simulink library "NeuroMuscularLibrary"  (R2019b)
settings: Solver=ode45  StartTime=0.0  StopTime=10.0  RelTol=1e-3  EnableMultiTasking=on
values from neighbouring files (symbols this model uses):
  a_18_19 = 116    [Prosthesis3R60Params.m]
  a_18_21 = 34    [Prosthesis3R60Params.m]
  a_2_3 = 18    [Prosthesis3R60Params.m]
  angle_offset = 0    [Prosthesis3R60Params.m]
  ankle_height = 0.08    [BodyMechParams.m]
  c = 0.05    [BodyMechParams.m]
  c_jointstop = 0.3 / (pi/180)    (= 17.1887338539)    [BodyMechParams.m]
  c_stance_comp_a0 = 885.0653    [Prosthesis3R60Params.m]
  c_stance_comp_a1 = 2.1443    [Prosthesis3R60Params.m]
  cg14 = 1/2*L14    (= 0.0475)    [Prosthesis3R60Params.m]
  cg25 = (5.45/11.05)*L25    (= 0.0379527149321)    [Prosthesis3R60Params.m]
  cg3 = (3.6/10.4)*L3    (= 0.0306346153846)    [Prosthesis3R60Params.m]
  d_fBall = 0.1    [BodyMechParams.m]
  d_fHeel = 0.05    [BodyMechParams.m]
  deltaLegAngleThr = 8*pi/180    (= 0.13962634016)    [CMGParams.m]
  DeltaThRef = 2e-3    (= 0.002)    [BodyMechParams.m]
  dt_visual = 0.001    [Prosthesis3R60Params.m]
  eref = 0.04    [BodyMechParams.m]
  Fmax = 4000    [MuscleEnergyTest.m]
  FmaxGLU = 1500    [BodyMechParams.m]
  footBallToAnkleDist = 0.16    [BodyMechParams.m]
  footBallToCenterDist = footLength/2    (= 0.1)    [BodyMechParams.m]
  footBallToHeelDist = footLength    (= 0.2)    [BodyMechParams.m]
  footCenterToCGDist = 0.14 - footBallToCenterDist    (= 0.04)    [BodyMechParams.m]
  footInertia = 0.005    [BodyMechParams.m]
  footLength = 0.2    [BodyMechParams.m]
  footMass = 1.25    [BodyMechParams.m]
  FT = 20    [MuscleEnergyTest.m]
  FT_GLU = 47.6    [BodyMechParams.m]
  g = 9.80665    [BodyMechParams.m]
  groundTheta = [atan(diff(groundZ)./diff(groundX)), 0]    [generateGround.m]
  groundZ = groundZ * stepSize/(largestStep+eps)    [generateGround.m]
  hatCenterToCGDist = 0.35 - hatHipToCenterDistLen    (= -0.05)    [BodyMechParams.m]
  hatHipToCenterDistLen = hatLength/2    (= 0.4)    [BodyMechParams.m]
  hatInertia = 3    [BodyMechParams.m]
  hatLeftHipToCenterDistWidth = .15    (= 0.15)    [BodyMechParams.m]
  hatLength = 0.8    [BodyMechParams.m]
  hatMass = 53.5    [BodyMechParams.m]
  hatThickness = 0.2    [BodyMechParams.m]
  hatWidth = 0.4    [BodyMechParams.m]
  J1011 = (4130)*1e-9    (= 4.13e-06)    [Prosthesis3R60Params.m]
  J1415 = (1.18*1e5)*1e-9    (= 0.000118)    [Prosthesis3R60Params.m]
  J18192021 = (6.86*1e4)*1e-9    (= 6.86e-05)    [Prosthesis3R60Params.m]
  J2526 = (3.59*1e4)*1e-9    (= 3.59e-05)    [Prosthesis3R60Params.m]
  J3467 = (25.96*1e4)*1e-9    (= 0.0002596)    [Prosthesis3R60Params.m]
  K = 5    [BodyMechParams.m]
  k_gn = k_gn/2    (= 39226.6)    [BodyMechParams.m]
  k_gt = k_gt/2    (= 39226.6)    [BodyMechParams.m]
  k_pressure = hatMass * g / DeltaThRef    (= 262327.8875)    [BodyMechParams.m]
  k_stance = 130000    [Prosthesis3R60Params.m]
  k_swing = 18750    [Prosthesis3R60Params.m]
  L0_stance = 0.08925    [Prosthesis3R60Params.m]
  L0_swing = 0.0896    [Prosthesis3R60Params.m]
  L10 = 7.9*1e-3    (= 0.0079)    [Prosthesis3R60Params.m]
  L11 = 3.3*1e-3    (= 0.0033)    [Prosthesis3R60Params.m]
  L14 = 95*1e-3    (= 0.095)    [Prosthesis3R60Params.m]
  L15 = 8.2*1e-3    (= 0.0082)    [Prosthesis3R60Params.m]
  L18 = 25.1*1e-3    (= 0.0251)    [Prosthesis3R60Params.m]
  L19 = 17.7*1e-3    (= 0.0177)    [Prosthesis3R60Params.m]
  L20 = 26*1e-3    (= 0.026)    [Prosthesis3R60Params.m]
  L21 = 1.7*1e-3    (= 0.0017)    [Prosthesis3R60Params.m]
  L25 = 76.95*1e-3    (= 0.07695)    [Prosthesis3R60Params.m]
  L26 = 2.8*1e-3    (= 0.0028)    [Prosthesis3R60Params.m]
  L3 = 88.5*1e-3    (= 0.0885)    [Prosthesis3R60Params.m]
  L4 = 1.7*1e-3    (= 0.0017)    [Prosthesis3R60Params.m]
  L6 = 40.25*1e-3    (= 0.04025)    [Prosthesis3R60Params.m]
  L7 = 14.9*1e-3    (= 0.0149)    [Prosthesis3R60Params.m]
  leg_l = [(thighLength - ankle_height/2) (shankLength - ankle_height/2)]    [BodyMechParams.m]
  legAngleSpeedMax = 10    [CMGParams.m]
  lopt = 0.055    [MuscleEnergyTest.m]
  loptBFSH = 0.12    [BodyMechParams.m]
  loptGAS = 0.05    [BodyMechParams.m]
  loptGLU = 0.11    [BodyMechParams.m]
  loptHAB = 0.09    [BodyMechParams.m]
  loptHAD = 0.10    (= 0.1)    [BodyMechParams.m]
  loptHAM = 0.10    (= 0.1)    [BodyMechParams.m]
  loptHFL = 0.11    [BodyMechParams.m]
  loptRF = 0.08    [BodyMechParams.m]
  loptSOL = 0.04    [BodyMechParams.m]
  loptTA = 0.06    [BodyMechParams.m]
  loptVAS = 0.08    [BodyMechParams.m]
  lslack = 0.245    [MuscleEnergyTest.m]
  lslackBFSH = 0.10    (= 0.1)    [BodyMechParams.m]
  lslackGAS = 0.40    (= 0.4)    [BodyMechParams.m]
  lslackGLU = 0.13    [BodyMechParams.m]
  lslackHAB = 0.07    [BodyMechParams.m]
  lslackHAD = 0.18    [BodyMechParams.m]
  lslackHAM = 0.31    [BodyMechParams.m]
  lslackHFL = 0.10    (= 0.1)    [BodyMechParams.m]
  lslackRF = 0.35    [BodyMechParams.m]
  lslackSOL = 0.26    [BodyMechParams.m]
  lslackTA = 0.24    [BodyMechParams.m]
  lslackVAS = 0.23    [BodyMechParams.m]
  m1011 = 49.5*1e-3    (= 0.0495)    [Prosthesis3R60Params.m]
  m1415 = 123.8*1e-3    (= 0.1238)    [Prosthesis3R60Params.m]
  m18192021 = 196.6*1e-3    (= 0.1966)    [Prosthesis3R60Params.m]
  m2526 = 58.3*1e-3    (= 0.0583)    [Prosthesis3R60Params.m]
  m3467 = 253.3*1e-3    (= 0.2533)    [Prosthesis3R60Params.m]
  mu_slide = 0.8    [BodyMechParams.m]
  mu_stick = 0.9    [BodyMechParams.m]
  N = 1.5    [BodyMechParams.m]    (also in cmaes.m = size(x,1); mergeCompareEnergyCosts.m = {S.name})
  phiKneeUpLimit = 5*pi/180    (= 0.0872664625997)    [BodyMechParams.m]
  phimaxGASa = (100-90)*pi/180    (= 0.174532925199)    [BodyMechParams.m]
  phimaxGASk = (180-140)*pi/180    (= 0.698131700798)    [BodyMechParams.m]
  phimaxRFk = (180-165)*pi/180    (= 0.261799387799)    [BodyMechParams.m]
  phimaxSOL = (100-90)*pi/180    (= 0.174532925199)    [BodyMechParams.m]
  phimaxTA = (80-90)*pi/180    (= -0.174532925199)    [BodyMechParams.m]
  phimaxVAS = (180-165)*pi/180    (= 0.261799387799)    [BodyMechParams.m]
  phirefBFSH = (180-160)*pi/180    (= 0.349065850399)    [BodyMechParams.m]
  phirefGASa = (80-90)*pi/180    (= -0.174532925199)    [BodyMechParams.m]
  phirefGASk = (180-165)*pi/180    (= 0.261799387799)    [BodyMechParams.m]
  phirefGLU = (120-180)*pi/180    (= -1.0471975512)    [BodyMechParams.m]
  phirefHAB = 10*pi/180    (= 0.174532925199)    [BodyMechParams.m]
  phirefHAD = 15*pi/180    (= 0.261799387799)    [BodyMechParams.m]
  phirefHAMh = (150-180)*pi/180    (= -0.523598775598)    [BodyMechParams.m]
  phirefHAMk = (180-180)*pi/180    (= 0)    [BodyMechParams.m]
  phirefHFL = (160-180)*pi/180    (= -0.349065850399)    [BodyMechParams.m]
  phirefRFh = (170-180)*pi/180    (= -0.174532925199)    [BodyMechParams.m]
  phirefRFk = (180-125)*pi/180    (= 0.959931088597)    [BodyMechParams.m]
  phirefSOL = (90-90)*pi/180    (= 0)    [BodyMechParams.m]
  ... (+64 more)
undefined symbols (not defined in the file or in its folder): ankleBackDriveGain, ankleCJointstop, ankleDgain, ankleFilterPID, ankleFilterSEA, ankleGearEff, ankleGearRatio, ankleIgain, ankleInitialAngle, ankleInputMass, ankleIntCoulomb, ankleIntDamping, ankleIntStatic, ankleParallelSpringDamping, ankleParallelSpringOffset, ankleParallelSpringStiffness, anklePgain, anklePlantarLimit, ankleSEADamping, ankleSEAStiffness, ankleTendonMass, ankleWMaxJointstop, D12_F, D12_S, D12_T, D12z_T, D13_F, D1G_F, D1G_HAT, D1G_S, D1G_T, D1Gy_F, DeltaS, DeltaSGLU, DeltaSHFL, dryFrictionDamping, dryFrictionStiffness, dryFrictionVelThresh, footMassp, FourBarL1, FourBarL3, GainDphiHATGLUst, GainDphiHATHABst, GainDphiHATHADst, GainDphiHATHFLst, GainFGASst, GainFGLUst, GainFHABst, GainFHAMst, GainFSOLst, GainFSOLTAst, GainFVASst, GainGAS, GainGLU, GainGLUswing, GainHAM, GainHAMHFL ... (+194)
libraries: sm_lib x332, nesl_utility x156, simulink x33, dspswit3 x30, $bdroot x19, simulink_extras x7
(part 14 of 15)

== system NeuroMuscularLibrary/RMHeel Cnt/3D Contact ==
  RefPt [m m m] : Inport
  nVec [m m m] : Inport  Port=2
  pVec [m m m] : Inport  Port=3
  vVec [m/s m/s m/s] : Inport  Port=4
  Contact! : EnablePort  StatesWhenEnabling=reset
  Friction Switch : Subsystem
  Kinetic Friction Model : Subsystem
  Logical Operator : Logic  Operator=NOT  AllPortsSameDT=off  OutDataTypeStr=boolean
  Static Friction Model : Subsystem
  Sum : Sum
  Sum1 : Sum
  FnVec [N N N] : Outport  OutputWhenDisabled=reset  InitialOutput=[0 0 0]
      settings: AttributesFormatString=when disabled: %<OutputWhenDisabled>
  FtVec [N N N] : Outport  Port=2  OutputWhenDisabled=reset  InitialOutput=[0 0 0]
      settings: AttributesFormatString=when disabled: %<OutputWhenDisabled>
  wires:
  pVec [m m m]/1 -> Static Friction Model/1(pos [m]), Kinetic Friction Model/2(pos [m m m])
  vVec [m/s m/s m/s]/1 -> Kinetic Friction Model/1(vel [m/s m/s m/s]), Static Friction Model/2(vel [m/s m/s m/s])
  Kinetic Friction Model/2(posFP [m m m]) -> Static Friction Model/4(posFP [m])
  Friction Switch/1(Stiction) -> Static Friction Model/Enable, Logical Operator/1
  Logical Operator/1 -> Kinetic Friction Model/Enable
  nVec [m m m]/1 -> Kinetic Friction Model/4(nVec [m m m])
  Kinetic Friction Model/4(Stiction!) -> Friction Switch/2(Stick!)
  Static Friction Model/1(F_n Stick [N N N]) -> Sum1/1
  Kinetic Friction Model/6(F_n Slide [N N N]) -> Sum1/2
  Kinetic Friction Model/5(F_t Slide [N N N]) -> Sum/2
  Static Friction Model/2(F_t Stick [N N N]) -> Sum/1
  Sum1/1 -> FnVec [N N N]/1  "F_nVec"
  Sum/1 -> FtVec [N N N]/1  "F_tVec"
  Static Friction Model/3(Sliding!) -> Friction Switch/1(Slide!)
  RefPt [m m m]/1 -> Kinetic Friction Model/3(RefPt [m m m])
  Kinetic Friction Model/3(nVec FP [m m m]) -> Static Friction Model/5(nVecFP [m m m])
  Kinetic Friction Model/1(RefPtFP [m m m]) -> Static Friction Model/3(RefPtFP [m m m])

== system NeuroMuscularLibrary/Swing Phase/Filtered Derivative ==
  In1 : Inport
  Filter Coeff : Gain  Gain=legAngleFilter
  Integrator : Integrator
  Sum4 : Sum  Inputs=|+-
  Out1 : Outport
  wires:
  Integrator/1 -> Sum4/2
  Sum4/1 -> Filter Coeff/1
  Filter Coeff/1 -> Integrator/1, Out1/1
  In1/1 -> Sum4/1

== system NeuroMuscularLibrary/Swing Phase/Knee Flex ==
  LegAngleSpeed : Inport
  Enable : EnablePort  StatesWhenEnabling=reset  ZeroCross=off
  " 4" : Gain  Gain=-kneeFlexGain
  Saturation : Saturate  UpperLimit=0  LowerLimit=-inf  ZeroCross=off
  tau : Outport  OutputWhenDisabled=reset  InitialOutput=0
  wires:
  LegAngleSpeed/1 -> Saturation/1
  " 4"/1 -> tau/1
  Saturation/1 -> " 4"/1

== system NeuroMuscularLibrary/Swing Phase/Knee Hold ==
  legAngleSpeed : Inport
  legAngle : Inport  Port=2
  legAngleTgt : Inport  Port=3
  kneeSpeed : Inport  Port=4
  Enable : EnablePort  StatesWhenEnabling=reset  ZeroCross=off
  " 5" : Gain  Gain=-kneeHoldGain1
  " 6" : Gain  Gain=-kneeHoldGain2
  Add4 : Sum
  Compare To Zero : simulink/Logic and Bit Operations/Compare To Zero  relop=>=  OutDataTypeStr=boolean  ZeroCross=off
  Compare To Zero1 : simulink/Logic and Bit Operations/Compare To Zero  relop=<  OutDataTypeStr=boolean  ZeroCross=off
  Product1 : Product
  Product2 : Product  Inputs=5
  Relational Operator : RelationalOperator  Operator=<  OutDataTypeStr=boolean  ZeroCross=off  RndMeth=Nearest
  Saturation : Saturate  UpperLimit=inf  LowerLimit=0
  Sum1 : Sum  Inputs=+-|
  Sum3 : Sum  Inputs=+-|
  tau : Outport  OutputWhenDisabled=reset  InitialOutput=0
  wires:
  Product1/1 -> Add4/1
  Saturation/1 -> Add4/2
  Add4/1 -> tau/1
  legAngleTgt/1 -> Sum1/2
  legAngle/1 -> Sum1/1
  legAngleSpeed/1 -> Relational Operator/2, Sum3/1
  Product2/1 -> Saturation/1
  Compare To Zero1/1 -> Product2/4
  Sum3/1 -> Product2/3
  Sum1/1 -> Product2/2
  " 6"/1 -> Product2/1
  kneeSpeed/1 -> Relational Operator/1, Compare To Zero1/1, Sum3/2, Compare To Zero/1, " 5"/1, " 6"/1  "knee speed"
  Compare To Zero/1 -> Product1/2
  " 5"/1 -> Product1/1
  Relational Operator/1 -> Product2/5

== system NeuroMuscularLibrary/Swing Phase/Knee Stop ==
  note: Knee Extend Torque
  legAngleSpeed : Inport
  legAngle : Inport  Port=2
  legAngleTgt : Inport  Port=3
  Leg Length : Inport  Port=4
  Extend? : Inport  Port=5
  Enable : EnablePort  StatesWhenEnabling=reset  ZeroCross=off
  Add : Sum
  Add5 : Sum  Inputs=-+
  Add6 : Sum  Inputs=+-
  Constant10 : Constant
  Constant11 : Constant  Value=legAngleSpeedMax
  Constant12 : Constant  Value=-kneeExtendGain
  Constant13 : Constant  Value=shankLength + thighLength
  Constant9 : Constant  Value=kneeStopGain
  Divide : Product  Inputs=*/
  Divide1 : Product  Inputs=***
  Product4 : Product  Inputs=5
  Relational Operator1 : RelationalOperator  Operator=<  OutDataTypeStr=boolean  ZeroCross=off  RndMeth=Nearest
  Relational Operator2 : RelationalOperator  Operator=<  OutDataTypeStr=boolean  ZeroCross=off  RndMeth=Nearest
  Sum2 : Sum  Inputs=++|
  Sum5 : Sum  Inputs=|-+
  leg angle Threshold : Constant  Value=deltaLegAngleThr
  tau : Outport  OutputWhenDisabled=reset  InitialOutput=0
  wires:
  Extend?/1 -> Divide1/1
  Leg Length/1 -> Sum5/1
  legAngleSpeed/1 -> Divide/1, Relational Operator2/1
  legAngle/1 -> Add5/1, Relational Operator1/1
  legAngleTgt/1 -> Sum2/1
  Add/1 -> tau/1
  Divide1/1 -> Add/2
  Sum5/1 -> Divide1/3
  Constant13/1 -> Sum5/2
  Constant12/1 -> Divide1/2
  Product4/1 -> Add/1
  Relational Operator2/1 -> Product4/5
  Relational Operator1/1 -> Product4/4
  Divide/1 -> Add6/2
  Constant10/1 -> Add6/1
  Add6/1 -> Product4/2
  Constant11/1 -> Divide/2, Relational Operator2/2
  Constant9/1 -> Product4/3
  Add5/1 -> Product4/1
  Sum2/1 -> Relational Operator1/2, Add5/2
  leg angle Threshold/1 -> Sum2/2

== system NeuroMuscularLibrary/Swing Phase/Wait 100 ms to enable ==
  In1 : Inport
  Clock : Clock
  Compare To Constant : simulink/Logic and Bit Operations/Compare To Constant  relop=>  const=.1  OutDataTypeStr=boolean  ZeroCross=off
  Product6 : Product
  Out1 : Outport
  wires:
  Product6/1 -> Out1/1
  Clock/1 -> Compare To Constant/1
  Compare To Constant/1 -> Product6/1
  In1/1 -> Product6/2

== system NeuroMuscularLibrary/Swing Phase (sagittal)/kneei_flexion from alpha ==
  note: Knee Phase i
  SBFSH : Inport
  Enable : EnablePort  StatesWhenEnabling=reset  ZeroCross=off
  SBFSH_Sw_ki : Outport  OutputWhenDisabled=reset  InitialOutput=0
  wires:
  SBFSH/1 -> SBFSH_Sw_ki/1

== system NeuroMuscularLibrary/Swing Phase (sagittal)/kneeii_damp and hold &kneeiii_leg stop &kneeiv_stance preparation ==
  note: Knee Phase i
  Target Leg Angle : Inport
  LceRF : Inport  Port=2
  LceHAM : Inport  Port=3
  VceHAM : Inport  Port=4
  VceVAS : Inport  Port=5
  VceBFSH : Inport  Port=6
  VceRF : Inport  Port=7
  LceHFL : Inport  Port=8
  LceGLU : Inport  Port=9
  LceVAS : Inport  Port=10
  Enable : EnablePort  StatesWhenEnabling=reset  ZeroCross=off
  " 1" : Gain  Gain=Sw_a2lopt_HAM
  " 9" : Gain  Gain=Sw_a2lopt_RF
  Compare To Constant : simulink/Logic and Bit Operations/Compare To Constant  relop=<=  const=0  OutDataTypeStr=uint8  ZeroCross=off
  Constant1 : Constant  Value=0  OutDataTypeStr=boolean
  Constant10 : Constant  Value=Sw_aRef_HAM
  Constant2 : Constant  Value=0  OutDataTypeStr=boolean
  Constant3 : Constant  Value=0  OutDataTypeStr=boolean
  Constant4 : Constant
  Constant5 : Constant
  Constant6 : Constant  Value=deltaLegAngleThr
  Constant8 : Constant  Value=Sw_aRef_RF
  Logical Operator : Logic  Operator=NOT  AllPortsSameDT=off  OutDataTypeStr=boolean
  Logical Operator1 : Logic  AllPortsSameDT=off  OutDataTypeStr=boolean
  Relational Operator : RelationalOperator  Operator=<=  OutDataTypeStr=boolean  ZeroCross=off  RndMeth=Nearest
  Relational Operator1 : RelationalOperator  OutDataTypeStr=boolean  ZeroCross=off  RndMeth=Nearest
  S-R Flip-Flop : simulink_extras/Flip Flops/S-R Flip-Flop  initial_condition=0
  S-R Flip-Flop1 : simulink_extras/Flip Flops/S-R Flip-Flop  initial_condition=0
  S-R Flip-Flop2 : simulink_extras/Flip Flops/S-R Flip-Flop  initial_condition=0
  Sum1 : Sum  Inputs=+-|  SaturateOnIntegerOverflow=on  InputSameDT=on  OutDataTypeStr=Inherit: Same as first input
  Sum2 : Sum  Inputs=++|  SaturateOnIntegerOverflow=on  InputSameDT=on  OutDataTypeStr=Inherit: Same as first input
  Sum3 : Sum  Inputs=|+-  SaturateOnIntegerOverflow=on  InputSameDT=on  OutDataTypeStr=Inherit: Same as first input
  Sum4 : Sum  Inputs=+-|  SaturateOnIntegerOverflow=on  InputSameDT=on  OutDataTypeStr=Inherit: Same as first input
  Sum5 : Sum  Inputs=++|  SaturateOnIntegerOverflow=on  InputSameDT=on  OutDataTypeStr=Inherit: Same as first input
  Terminator : Terminator
  Terminator1 : Terminator
  Terminator2 : Terminator
  kneeii_damp and hold : Subsystem  TreatAsAtomicUnit=on
  kneeiii_leg stop : Subsystem  TreatAsAtomicUnit=on
  kneeiv_stance preparation : Subsystem  TreatAsAtomicUnit=on
  SRF_Sw_kii : Outport  OutputWhenDisabled=reset  InitialOutput=0
  SBFSH_Sw_kii : Outport  Port=2  OutputWhenDisabled=reset  InitialOutput=0
  SHAM_Sw_kiii : Outport  Port=3  OutputWhenDisabled=reset  InitialOutput=0
  SBFSH_Sw_kiii : Outport  Port=4  OutputWhenDisabled=reset  InitialOutput=0
  SGAS_Sw_kiii : Outport  Port=5  OutputWhenDisabled=reset  InitialOutput=0
  SHFL_Sw_kiv : Outport  Port=6  OutputWhenDisabled=reset  InitialOutput=0
  SGLU_Sw_kiv : Outport  Port=7  OutputWhenDisabled=reset  InitialOutput=0
  SVAS_Sw_kiv : Outport  Port=8  OutputWhenDisabled=reset  InitialOutput=0
  wires:
  Constant1/1 -> S-R Flip-Flop/2
  S-R Flip-Flop/2 -> Terminator/1
  Relational Operator/1 -> S-R Flip-Flop/1
  Constant2/1 -> S-R Flip-Flop1/2
  S-R Flip-Flop1/2 -> Terminator1/1
  Relational Operator1/1 -> S-R Flip-Flop1/1
  Constant3/1 -> S-R Flip-Flop2/2
  S-R Flip-Flop2/2 -> Terminator2/1
  Logical Operator1/1 -> S-R Flip-Flop2/1
  S-R Flip-Flop/1 -> Logical Operator/1
  S-R Flip-Flop1/1 -> kneeiii_leg stop/Enable, Logical Operator1/1
  S-R Flip-Flop2/1 -> kneeiv_stance preparation/Enable
  kneeii_damp and hold/1(SRF_Sw_kii) -> SRF_Sw_kii/1
  kneeii_damp and hold/2(SBFSH_Sw_kii) -> SBFSH_Sw_kii/1
  kneeiii_leg stop/1(SHAM_Sw_kiii) -> SHAM_Sw_kiii/1
  kneeiii_leg stop/2(SBFSH_Sw_kiii) -> SBFSH_Sw_kiii/1
  kneeiii_leg stop/3(SGAS_Sw_kiii) -> SGAS_Sw_kiii/1
  kneeiv_stance preparation/1(SHFL_Sw_kiv) -> SHFL_Sw_kiv/1
  kneeiv_stance preparation/2(SGLU_Sw_kiv) -> SGLU_Sw_kiv/1
  kneeiv_stance preparation/3(SVAS_Sw_kiv) -> SVAS_Sw_kiv/1
  Sum3/1 -> " 9"/1
  Constant4/1 -> Sum5/2
  " 9"/1 -> Sum5/1
  Target Leg Angle/1 -> kneeiv_stance preparation/1(Target Leg Angle), kneeiii_leg stop/1(Target Leg Angle), kneeii_damp and hold/1(Target Leg Angle), Sum3/1, Sum2/1
  Sum5/1 -> Relational Operator/2  "lceOffRF"
  LceRF/1 -> Relational Operator/1, kneeii_damp and hold/5(LceRF)
  Logical Operator/1 -> kneeii_damp and hold/Enable
  Sum2/1 -> Sum1/1  "a_thr"
  Sum1/1 -> " 1"/1
  Constant5/1 -> Sum4/1
  " 1"/1 -> Sum4/2
  Sum4/1 -> Relational Operator1/2  "lceOffHAM"
  LceHAM/1 -> kneeiii_leg stop/2(LceHAM), Relational Operator1/1  "LceHAM"
  Compare To Constant/1 -> Logical Operator1/2
  VceHAM/1 -> Compare To Constant/1
  VceBFSH/1 -> kneeii_damp and hold/3(VceBFSH)
  VceRF/1 -> kneeii_damp and hold/4(VceRF)
  LceHFL/1 -> kneeiv_stance preparation/2(LceHFL)
  LceGLU/1 -> kneeiv_stance preparation/3(LceGLU)
  LceVAS/1 -> kneeiv_stance preparation/4(LceVAS)
  VceVAS/1 -> kneeii_damp and hold/2(VceVAS)
  Constant10/1 -> Sum1/2
  Constant6/1 -> Sum2/2
  Constant8/1 -> Sum3/2

== system NeuroMuscularLibrary/Swing Phase Hip muscle/Filtered Derivative ==
  In1 : Inport
  Filter Coeff : Gain  Gain=legAngleFilter
  Integrator : Integrator
  Sum4 : Sum  Inputs=|+-
  Out1 : Outport
  wires:
  In1/1 -> Sum4/1
  Filter Coeff/1 -> Out1/1, Integrator/1
  Sum4/1 -> Filter Coeff/1
  Integrator/1 -> Sum4/2

== system NeuroMuscularLibrary/Swing Phase Hip muscle/Knee Flex ==
  LegAngleSpeed : Inport
  Enable : EnablePort  StatesWhenEnabling=reset  ZeroCross=off
  " 4" : Gain  Gain=-kneeFlexGain
  Saturation : Saturate  UpperLimit=0  LowerLimit=-inf  ZeroCross=off
  tau : Outport  OutputWhenDisabled=reset  InitialOutput=0
  wires:
  Saturation/1 -> " 4"/1
  " 4"/1 -> tau/1
  LegAngleSpeed/1 -> Saturation/1

== system NeuroMuscularLibrary/Swing Phase Hip muscle/Knee Hold ==
  legAngleSpeed : Inport
  legAngle : Inport  Port=2
  legAngleTgt : Inport  Port=3
  kneeSpeed : Inport  Port=4
  Enable : EnablePort  StatesWhenEnabling=reset  ZeroCross=off
  " 5" : Gain  Gain=-kneeHoldGain1
  " 6" : Gain  Gain=-kneeHoldGain2
  Add4 : Sum
  Compare To Zero : simulink/Logic and Bit Operations/Compare To Zero  relop=>=  OutDataTypeStr=boolean  ZeroCross=off
  Compare To Zero1 : simulink/Logic and Bit Operations/Compare To Zero  relop=<  OutDataTypeStr=boolean  ZeroCross=off
  Product1 : Product
  Product2 : Product  Inputs=5
  Relational Operator : RelationalOperator  Operator=<  OutDataTypeStr=boolean  ZeroCross=off  RndMeth=Nearest
  Saturation : Saturate  UpperLimit=inf  LowerLimit=0
  Sum1 : Sum  Inputs=+-|
  Sum3 : Sum  Inputs=+-|
  tau : Outport  OutputWhenDisabled=reset  InitialOutput=0
  wires:
  Relational Operator/1 -> Product2/5
  " 5"/1 -> Product1/1
  Compare To Zero/1 -> Product1/2
  kneeSpeed/1 -> " 6"/1, " 5"/1, Compare To Zero/1, Sum3/2, Compare To Zero1/1, Relational Operator/1  "knee speed"
  " 6"/1 -> Product2/1
  Sum1/1 -> Product2/2
  Sum3/1 -> Product2/3
  Compare To Zero1/1 -> Product2/4
  Product2/1 -> Saturation/1
  legAngleSpeed/1 -> Sum3/1, Relational Operator/2
  legAngle/1 -> Sum1/1
  legAngleTgt/1 -> Sum1/2
  Add4/1 -> tau/1
  Saturation/1 -> Add4/2
  Product1/1 -> Add4/1

== system NeuroMuscularLibrary/Swing Phase Hip muscle/Knee Stop ==
  note: Knee Extend Torque
  legAngleSpeed : Inport
  legAngle : Inport  Port=2
  legAngleTgt : Inport  Port=3
  Leg Length : Inport  Port=4
  Extend? : Inport  Port=5
  Enable : EnablePort  StatesWhenEnabling=reset  ZeroCross=off
  Add : Sum
  Add5 : Sum  Inputs=-+
  Add6 : Sum  Inputs=+-
  Constant10 : Constant
  Constant11 : Constant  Value=legAngleSpeedMax
  Constant12 : Constant  Value=-kneeExtendGain
  Constant13 : Constant  Value=shankLength + thighLength
  Constant9 : Constant  Value=kneeStopGain
  Divide : Product  Inputs=*/
  Divide1 : Product  Inputs=***
  Product4 : Product  Inputs=5
  Relational Operator1 : RelationalOperator  Operator=<  OutDataTypeStr=boolean  ZeroCross=off  RndMeth=Nearest
  Relational Operator2 : RelationalOperator  Operator=<  OutDataTypeStr=boolean  ZeroCross=off  RndMeth=Nearest
  Sum2 : Sum  Inputs=++|
  Sum5 : Sum  Inputs=|-+
  leg angle Threshold : Constant  Value=deltaLegAngleThr
  tau : Outport  OutputWhenDisabled=reset  InitialOutput=0
  wires:
  leg angle Threshold/1 -> Sum2/2
  Sum2/1 -> Add5/2, Relational Operator1/2
  Add5/1 -> Product4/1
  Constant9/1 -> Product4/3
  Constant11/1 -> Relational Operator2/2, Divide/2
  Add6/1 -> Product4/2
  Constant10/1 -> Add6/1
  Divide/1 -> Add6/2
  Relational Operator1/1 -> Product4/4
  Relational Operator2/1 -> Product4/5
  Product4/1 -> Add/1
  Constant12/1 -> Divide1/2
  Constant13/1 -> Sum5/2
  Sum5/1 -> Divide1/3
  Divide1/1 -> Add/2
  Add/1 -> tau/1
  legAngleTgt/1 -> Sum2/1
  legAngle/1 -> Relational Operator1/1, Add5/1
  legAngleSpeed/1 -> Relational Operator2/1, Divide/1
  Leg Length/1 -> Sum5/1
  Extend?/1 -> Divide1/1

== system NeuroMuscularLibrary/Swing Phase Hip muscle/Wait 100 ms to enable ==
  In1 : Inport
  Clock : Clock
  Compare To Constant : simulink/Logic and Bit Operations/Compare To Constant  relop=>  const=.1  OutDataTypeStr=boolean  ZeroCross=off
  Product6 : Product
  Out1 : Outport
  wires:
  In1/1 -> Product6/2
  Compare To Constant/1 -> Product6/1
  Clock/1 -> Compare To Constant/1
  Product6/1 -> Out1/1

== system NeuroMuscularLibrary/ThighSong/Sensor Sheet ==
  note: Inner Segment Pressure Sheet
  FB Gain1 : Gain  Gain=1/DeltaThRef  SaturateOnIntegerOverflow=on  OutDataTypeStr=Inherit: Same as input  ParamDataTypeStr=Inherit: Same as input
  Gain1 : Gain  Gain=-1
  Gain3 : Gain  Gain=k_pressure
  Gain4 : Gain  Gain=1/v_max_pressure
  Mux1 : Mux  Inputs=2
  PS-Simulink Converter : nesl_utility/PS-Simulink Converter  PhysicalDomain=network_engine_domain  SubClassName=ps_output  LeftPortType=input  RightPortType=output  PseudoPeriodic=off  Frequencies=[]  Unit=1  AffineConversion=off
  PS-Simulink Converter1 : nesl_utility/PS-Simulink Converter  PhysicalDomain=network_engine_domain  SubClassName=ps_output  LeftPortType=input  RightPortType=output  PseudoPeriodic=off  Frequencies=[]  Unit=1  AffineConversion=off
  Pressure Sheet Reaction Force : Fcn  Expr=-u(1) * (1+sgn(u(1))*u(2))
  Prismatic Joint : sm_lib/Joints/Prismatic Joint  JointMode=Normal  SenseConstraintForce=off  SenseConstraintForceX=off  SenseConstraintForceY=off  SenseConstraintForceZ=off  SenseConstraintTorque=off  SenseConstraintTorqueX=off  SenseConstraintTorqueY=off  SenseConstraintTorqueZ=off  SenseTotalForce=off  SenseTotalForceX=off  SenseTotalForceY=off  SenseTotalForceZ=off  SenseTotalTorque=off  SenseTotalTorqueX=off  SenseTotalTorqueY=off  SenseTotalTorqueZ=off  CompositeWrenchDir=FollowerOnBase  CompositeWrenchFrame=BaseFrame  EquilibriumPosition=0  EquilibriumPositionUnits=m  SpringStiffness=0  SpringStiffnessUnits=N/m  DampingCoefficient=0  DampingCoefficientUnits=N/(m/s)  TorqueActuationMode=InputTorque  MotionActuationMode=ComputedMotion  SensePosition=on  SenseVelocity=on  SenseAcceleration=off  SenseTorqueForce=off  SenseLowerLimitTorqueForce=off  SenseUpperLimitTorqueForce=off  LowerLimitSpecify=off  LowerLimitBound=-1  LowerLimitBoundUnits=m  LowerLimitStiffness=1e6  LowerLimitStiffnessUnits=N/m  LowerLimitDamping=1e3  LowerLimitDampingUnits=N/(m/s)  LowerLimitTransitionRegionWidth=1e-4  LowerLimitTransitionRegionWidthUnits=m  UpperLimitSpecify=off  UpperLimitBound=1  UpperLimitBoundUnits=m  UpperLimitStiffness=1e6  UpperLimitStiffnessUnits=N/m  UpperLimitDamping=1e3  UpperLimitDampingUnits=N/(m/s)  UpperLimitTransitionRegionWidth=1e-4  UpperLimitTransitionRegionWidthUnits=m  PositionTargetSpecify=on  PositionTargetPriority=High  PositionTargetValue=0  PositionTargetValueUnits=m  VelocityTargetSpecify=on  VelocityTargetPriority=High  VelocityTargetValue=0  VelocityTargetValueUnits=m/s
  Saturation11 : Saturate  UpperLimit=inf  LowerLimit=0  ZeroCross=off
  Simulink-PS Converter : nesl_utility/Simulink-PS Converter  PhysicalDomain=network_engine_domain  SubClassName=ps_input  LeftPortType=input  RightPortType=output  PseudoPeriodic=off  Frequencies=[]  NoiseDistribution=none  NoiseParameters=[]  Unit=1  AffineConversion=off  FilteringAndDerivatives=zero  SimscapeFilterOrder=1  InputFilterTimeConstant=0.001  UdotUserProvided=1
  Y-up TO Z-up : sm_lib/Frames and Transforms/Rigid Transform  TranslationMethod=None  TranslationStandardOffset=0  TranslationLengthUnit=m  TranslationStandardAxis=+Z  TranslationCartesianOffset=[0 0 0]  TranslationROffset=0  TranslationROffsetUnits=m  TranslationZOffset=0  TranslationZOffsetUnits=m  TranslationThetaOffset=0  TranslationThetaOffsetUnits=deg  RotationMethod=AlignedAxes  RotationAngleUnits=deg  RotationStandardAxis=+Z  RotationAngle=0  RotationArbitraryAxis=[0 0 1]  FollAlignAxisA=+X  BaseAlignAxisA=+X  FollAlignAxisB=+Z  BaseAlignAxisB=+Y  RotationSequenceAxes=FollowerAxes  RotationSequence=XYX  RotationSequenceAngles=[0 0 0]  RotationSequenceAnglesUnits=deg  RotationMatrix=[1 0 0; 0 1 0; 0 0 1]
  Z-up TO Y-up : sm_lib/Frames and Transforms/Rigid Transform  TranslationMethod=None  TranslationStandardOffset=0  TranslationLengthUnit=m  TranslationStandardAxis=+Z  TranslationCartesianOffset=[0 0 0]  TranslationROffset=0  TranslationROffsetUnits=m  TranslationZOffset=0  TranslationZOffsetUnits=m  TranslationThetaOffset=0  TranslationThetaOffsetUnits=deg  RotationMethod=AlignedAxes  RotationAngleUnits=deg  RotationStandardAxis=+Z  RotationAngle=0  RotationArbitraryAxis=[0 0 1]  FollAlignAxisA=+X  BaseAlignAxisA=+X  FollAlignAxisB=+Y  BaseAlignAxisB=+Z  RotationSequenceAxes=FollowerAxes  RotationSequence=XYX  RotationSequenceAngles=[0 0 0]  RotationSequenceAnglesUnits=deg  RotationMatrix=[1 0 0; 0 1 0; 0 0 1]
  smooth : TransferFcn  Denominator=[0.02 1]
  Lower thigh : PMIOPort  Side=Left
  Upper thigh : PMIOPort  Port=2  Side=Right
  dx : Outport
  Thigh Fx : Outport  Port=2
  wires:
  PS-Simulink Converter/1 -> Gain1/1, Gain3/1  "position"
  PS-Simulink Converter1/1 -> Gain4/1  "velocity"
  Mux1/1 -> Pressure Sheet Reaction Force/1
  Gain3/1 -> Mux1/1
  Gain4/1 -> Mux1/2
  Pressure Sheet Reaction Force/1 -> Simulink-PS Converter/1
  FB Gain1/1 -> Thigh Fx/1
  smooth/1 -> Saturation11/1
  Saturation11/1 -> FB Gain1/1
  Gain1/1 -> smooth/1, dx/1
  connections:
  Prismatic Joint/LConn1 -- Y-up TO Z-up/RConn1
  Prismatic Joint/RConn1 -- Z-up TO Y-up/LConn1
  Prismatic Joint/LConn2 -- Simulink-PS Converter/RConn1
  Prismatic Joint/RConn2 -- PS-Simulink Converter/LConn1
  Prismatic Joint/RConn3 -- PS-Simulink Converter1/LConn1
  Y-up TO Z-up/LConn1 -- Lower thigh/RConn1
  Upper thigh/RConn1 -- Z-up TO Y-up/RConn1

== system NeuroMuscularLibrary/Full Prosthesis/Ankle  Joint/Ankle Plantarflexion Limit ==
  note: Knee/Hip Joint Limits
  phi [rad] : Inport
  dphi [rad/s] : Inport  Port=2
  Compare To Constant : simulink/Logic and Bit Operations/Compare To Constant  relop=<  const=1.0  OutDataTypeStr=boolean  ZeroCross=off
  Compare To Zero : simulink/Logic and Bit Operations/Compare To Zero  relop=>  OutDataTypeStr=boolean  ZeroCross=off
  Constant : Constant
  Gain : Gain  Gain=-1
  Gain1 : Gain  Gain=ext
  Gain2 : Gain  Gain=-ext
  Gain3 : Gain  Gain=c_jointstop
  Gain4 : Gain  Gain=1/w_max_jointstop
  Gain5 : Gain  Gain=ext
  Product : Product  Inputs=4
  Sum : Sum  Inputs=|+-
  Sum1 : Sum  Inputs=|+-
  overextension angle : Constant  Value=phiUpLimit
  M_stop [Nm] : Outport
  wires:
  Sum/1 -> Gain3/1
  Gain1/1 -> Compare To Zero/1, Gain/1
  Gain3/1 -> Gain1/1
  dphi [rad/s]/1 -> Gain4/1
  overextension angle/1 -> Sum/2
  phi [rad]/1 -> Sum/1
  Gain4/1 -> Gain2/1
  Gain2/1 -> Compare To Constant/1, Sum1/2
  Gain5/1 -> M_stop [Nm]/1
  Constant/1 -> Sum1/1
  Gain/1 -> Product/1
  Sum1/1 -> Product/2
  Compare To Constant/1 -> Product/3
  Compare To Zero/1 -> Product/4
  Product/1 -> Gain5/1

== system NeuroMuscularLibrary/Full Prosthesis/Ankle Motor/Friction ==
  Velocity : Inport
  Abs : Abs  ZeroCross=off
  Add : Sum  Inputs=+++
  Divide : Product  Inputs=*/*
  Gain : Gain  Gain=sigma0
  Gain1 : Gain  Gain=sigma1
  Gain2 : Gain  Gain=Fv
  Gain3 : Gain  Gain=-1
  Integrator : Integrator  ZeroCross=off
  Subtract : Sum  Inputs=+-
  g(v) : Fcn  Expr=(Fc + (Fs - Fc)*exp(-(u/v_s)^2))/sigma0
  Friction Force : Outport
  wires:
  Gain2/1 -> Add/1
  Gain/1 -> Add/2
  Gain1/1 -> Add/3
  Gain3/1 -> Friction Force/1
  Add/1 -> Gain3/1
  Integrator/1 -> Gain/1, Divide/3  "z"
  g(v)/1 -> Divide/2
  Subtract/1 -> Gain1/1, Integrator/1  "dz/dt"
  Divide/1 -> Subtract/2
  Abs/1 -> Divide/1
  Velocity/1 -> Subtract/1, Abs/1, g(v)/1, Gain2/1

== system NeuroMuscularLibrary/Full Prosthesis/Ankle Motor/Motor Dynamics ==
  Voltage : Inport
  Speed : Inport  Port=2
  1/Inductance : Gain  Gain=1/motorInductance
  Add : Sum  Inputs=+--
  Integrator : Integrator
  Resistance : Gain  Gain=motorResistance
  Saturation : Saturate  UpperLimit=motorMaxCurrent  LowerLimit=-motorMaxCurrent  ZeroCross=off
  Torsional Constant : Gain  Gain=motorTorsionalConst
  back EMF : Gain  Gain=motorBackEMF
  Torque : Outport
  wires:
  Integrator/1 -> Saturation/1
  Saturation/1 -> Torsional Constant/1, Resistance/1  "Current"
  Resistance/1 -> Add/2
  back EMF/1 -> Add/3
  1/Inductance/1 -> Integrator/1  "di/dt"
  Add/1 -> 1/Inductance/1
  Speed/1 -> back EMF/1
  Torsional Constant/1 -> Torque/1  "Torque"
  Voltage/1 -> Add/1

== system NeuroMuscularLibrary/Full Prosthesis/Ankle SEA Control/4 bar ratio ==
  Ankle Input Angle : Inport
  Tendon Angle : Inport  Port=2
  Ankle Angle : Inport  Port=3
  Add : Sum  Inputs=--+
  Bias1 : Bias  Bias=-atan(16.3/81)
  Bias3 : Bias  Bias=5*pi/2
  Divide : Product  Inputs=*/
  Gain1 : Gain  Gain=-1
  Gain2 : Gain  Gain=-1
  Gain3 : Gain  Gain=-FourBarL3/FourBarL1
  Gain4 : Gain  Gain=-1
  Trigonometric Function : Trigonometry
  Trigonometric Function1 : Trigonometry
  ratio : Outport
  wires:
  Gain1/1 -> Bias3/1
  Bias1/1 -> Add/3
  Bias3/1 -> Trigonometric Function1/1, Add/2
  Ankle Angle/1 -> Gain4/1
  Gain4/1 -> Bias1/1
  Gain3/1 -> ratio/1  "4 bar ratio"
  Gain2/1 -> Add/1
  Ankle Input Angle/1 -> Gain2/1
  Add/1 -> Trigonometric Function/1
  Tendon Angle/1 -> Gain1/1
  Trigonometric Function/1 -> Divide/1
  Trigonometric Function1/1 -> Divide/2
  Divide/1 -> Gain3/1

== system NeuroMuscularLibrary/Full Prosthesis/Ankle SEA Control/Feed Forward ==
  Motor Speed : Inport
  Load Acceleration : Inport  Port=2
  Desired Actuator Torque : Inport  Port=3
  1/n : Gain  Gain=1/ankleGearRatio
  Back EMF : Gain  Gain=motorBackEMF
  Filter Coeff : Gain  Gain=ankleFilterSEA
  Integrator : Integrator
  K_b*J_m*n : Gain  Gain=ankleBackDriveGain*motorRotorInertia*ankleGearRatio
  R/K_tau : Gain  Gain=motorResistance/motorTorsionalConst
  Sum : Sum  Inputs=+-|
  Sum1 : Sum  Inputs=|+-
  Sum2 : Sum
  Computed Motor Voltage : Outport
  wires:
  Filter Coeff/1 -> Integrator/1
  Sum1/1 -> Filter Coeff/1
  Integrator/1 -> Sum1/2, K_b*J_m*n/1  "Filtered Accel"
  Load Acceleration/1 -> Sum1/1
  Back EMF/1 -> Sum/1
  Sum2/1 -> R/K_tau/1
  R/K_tau/1 -> Sum/2
  Motor Speed/1 -> Back EMF/1
  Desired Actuator Torque/1 -> 1/n/1
  1/n/1 -> Sum2/2
  K_b*J_m*n/1 -> Sum2/1
  Sum/1 -> Computed Motor Voltage/1

== system NeuroMuscularLibrary/Full Prosthesis/Knee Joint/Friction ==
  Velocity : Inport
  Abs : Abs  ZeroCross=off
  Add : Sum  Inputs=+++
  Divide : Product  Inputs=*/*
  Gain : Gain  Gain=sigma0
  Gain1 : Gain  Gain=sigma1
  Gain2 : Gain  Gain=Fv
  Gain3 : Gain  Gain=-1
  Integrator : Integrator  ZeroCross=off
  Subtract : Sum  Inputs=+-
  g(v) : Fcn  Expr=(Fc + (Fs - Fc)*exp(-(u/v_s)^2))/sigma0
  Friction Force : Outport
  wires:
  Gain2/1 -> Add/1
  Gain/1 -> Add/2
  Gain1/1 -> Add/3
  Gain3/1 -> Friction Force/1
  Add/1 -> Gain3/1
  Integrator/1 -> Gain/1, Divide/3  "z"
  g(v)/1 -> Divide/2
  Subtract/1 -> Gain1/1, Integrator/1  "dz/dt"
  Divide/1 -> Subtract/2
  Abs/1 -> Divide/1
  Velocity/1 -> Subtract/1, Abs/1, g(v)/1, Gain2/1

== system NeuroMuscularLibrary/Full Prosthesis/Knee Joint/Knee Plantarflexion Limit ==
  note: Knee/Hip Joint Limits
  phi [rad] : Inport
  dphi [rad/s] : Inport  Port=2
  Compare To Constant : simulink/Logic and Bit Operations/Compare To Constant  relop=<  const=1.0  OutDataTypeStr=boolean  ZeroCross=off
  Compare To Zero : simulink/Logic and Bit Operations/Compare To Zero  relop=>  OutDataTypeStr=boolean  ZeroCross=off
  Constant : Constant
  Gain : Gain  Gain=-1
  Gain1 : Gain  Gain=ext
  Gain2 : Gain  Gain=-ext
  Gain3 : Gain  Gain=c_jointstop
  Gain4 : Gain  Gain=1/w_max_jointstop
  Gain5 : Gain  Gain=ext
  Product : Product  Inputs=4
  Sum : Sum  Inputs=|+-
  Sum1 : Sum  Inputs=|+-
  overextension angle : Constant  Value=phiUpLimit
  M_stop [Nm] : Outport
  wires:
  Product/1 -> Gain5/1
  Compare To Zero/1 -> Product/4
  Compare To Constant/1 -> Product/3
  Sum1/1 -> Product/2
  Gain/1 -> Product/1
  Constant/1 -> Sum1/1
  Gain5/1 -> M_stop [Nm]/1
  Gain2/1 -> Sum1/2, Compare To Constant/1
  Gain4/1 -> Gain2/1
  phi [rad]/1 -> Sum/1
  overextension angle/1 -> Sum/2
  dphi [rad/s]/1 -> Gain4/1
  Gain3/1 -> Gain1/1
  Gain1/1 -> Gain/1, Compare To Zero/1
  Sum/1 -> Gain3/1

== system NeuroMuscularLibrary/Full Prosthesis/Knee Motor/Friction ==
  Velocity : Inport
  Abs : Abs  ZeroCross=off
  Add : Sum  Inputs=+++
  Divide : Product  Inputs=*/*
  Gain : Gain  Gain=sigma0
  Gain1 : Gain  Gain=sigma1
  Gain2 : Gain  Gain=Fv
  Gain3 : Gain  Gain=-1
  Integrator : Integrator  ZeroCross=off
  Subtract : Sum  Inputs=+-
  g(v) : Fcn  Expr=(Fc + (Fs - Fc)*exp(-(u/v_s)^2))/sigma0
  Friction Force : Outport
  wires:
  Gain2/1 -> Add/1
  Gain/1 -> Add/2
  Gain1/1 -> Add/3
  Gain3/1 -> Friction Force/1
  Add/1 -> Gain3/1
  Integrator/1 -> Gain/1, Divide/3  "z"
  g(v)/1 -> Divide/2
  Subtract/1 -> Gain1/1, Integrator/1  "dz/dt"
  Divide/1 -> Subtract/2
  Abs/1 -> Divide/1
  Velocity/1 -> Subtract/1, Abs/1, g(v)/1, Gain2/1

== system NeuroMuscularLibrary/Full Prosthesis/Knee Motor/Motor Dynamics ==
  Voltage : Inport
  Speed : Inport  Port=2
  1/Inductance : Gain  Gain=1/motorInductance
  Add : Sum  Inputs=+--
  Integrator : Integrator
  Resistance : Gain  Gain=motorResistance
  Saturation : Saturate  UpperLimit=motorMaxCurrent  LowerLimit=-motorMaxCurrent  ZeroCross=off
  Torsional Constant : Gain  Gain=motorTorsionalConst
  back EMF : Gain  Gain=motorBackEMF
  Torque : Outport
  wires:
  Integrator/1 -> Saturation/1
  Saturation/1 -> Torsional Constant/1, Resistance/1  "Current"
  Resistance/1 -> Add/2
  back EMF/1 -> Add/3
  1/Inductance/1 -> Integrator/1  "di/dt"
  Add/1 -> 1/Inductance/1
  Speed/1 -> back EMF/1
  Torsional Constant/1 -> Torque/1  "Torque"
  Voltage/1 -> Add/1

== system NeuroMuscularLibrary/Full Prosthesis/Knee SEA Control/Feed Forward ==
  Motor Speed : Inport
  Load Acceleration : Inport  Port=2
  Desired Torque : Inport  Port=3
  1/n : Gain  Gain=1/kneeGearRatio
  Back EMF : Gain  Gain=motorBackEMF
  Filter Coeff : Gain  Gain=kneeFilterSEA
  Integrator : Integrator
  K_b*J_m*n : Gain  Gain=kneeBackDriveGain*motorRotorInertia*kneeGearRatio
  R/K_tau : Gain  Gain=motorResistance/motorTorsionalConst
  Sum : Sum  Inputs=+-|
  Sum1 : Sum  Inputs=|+-
  Sum2 : Sum
  Computed Motor Voltage : Outport
  wires:
  Filter Coeff/1 -> Integrator/1
  Sum1/1 -> Filter Coeff/1
  Integrator/1 -> Sum1/2, K_b*J_m*n/1  "Filtered Accel"
  Load Acceleration/1 -> Sum1/1
  Back EMF/1 -> Sum/1
  Sum2/1 -> R/K_tau/1
  R/K_tau/1 -> Sum/2
  Motor Speed/1 -> Back EMF/1
  Desired Torque/1 -> 1/n/1
  1/n/1 -> Sum2/2
  K_b*J_m*n/1 -> Sum2/1
  Sum/1 -> Computed Motor Voltage/1

== system NeuroMuscularLibrary/Ground Contact Model/2D Contact/Friction Switch ==
  note: Static/Kinetic Friction Switch
  Slide! : Inport
  Stick! : Inport  Port=2
  Memory : Memory
  S-R Flip-Flop : simulink_extras/Flip Flops/S-R Flip-Flop  initial_condition=0
  Terminator : Terminator
  Stiction : Outport
  wires:
  Memory/1 -> Stiction/1
  Slide!/1 -> S-R Flip-Flop/2
  Stick!/1 -> S-R Flip-Flop/1
  S-R Flip-Flop/2 -> Terminator/1
  S-R Flip-Flop/1 -> Memory/1

== system NeuroMuscularLibrary/Ground Contact Model/2D Contact/Kinetic Friction Model ==
  note: Tangential Ground Friction
  note: Normal Ground Friction
  note: Sliding Limit Detector
  note: Footpoint Determiner
  note: Kinetic Friction Model
  vel [m/s m/s] : Inport
  pos [m m] : Inport  Port=2
  RefPt [m m] : Inport  Port=3
  nVec [m m] : Inport  Port=4
  Enable : EnablePort  StatesWhenEnabling=reset  ZeroCross=off
  Add : Sum  Inputs=-+
  Compare To Constant : simulink/Logic and Bit Operations/Compare To Constant  relop=<  const=1  OutDataTypeStr=boolean
  Constant : Constant  Value=vLimit
  Constant2 : Constant
  FixPt Relational Operator : RelationalOperator  Operator=>  OutDataTypeStr=boolean  ZeroCross=off  RndMeth=Nearest
  Gain3 : Gain  Gain=k_gn
  Gain4 : Gain  Gain=1/v_gn_max
  Memory : Memory
  Negative : simulink/Logic and Bit Operations/Compare To Zero  relop=<  OutDataTypeStr=boolean
  Product : Product  RndMeth=Zero
  Product1 : Product  RndMeth=Zero
  Product2 : Product  Inputs=3
  Scope : Scope
  Sum : Sum  Inputs=|+-
  Vector Norm : Subsystem
  d_n : DotProduct  InputSameDT=on  OutDataTypeStr=Inherit: Inherit via internal rule
  qnVec : Sum  Inputs=-+
  reverse direction : Gain  Gain=-1
  sliding friction coefficient : Gain  Gain=mu_slide
  tVec : Product  Inputs=*/  RndMeth=Zero
  v_n : DotProduct  InputSameDT=on  OutDataTypeStr=Inherit: Inherit via internal rule
  v_nVec : Product  RndMeth=Zero
  v_tVec : Sum  Inputs=-+|
  RefPtFP [m m] : Outport  InitialOutput=[0 0]
      settings: AttributesFormatString=initial = '%<InitialOutput>'\nwhen disabled = '%<OutputWhenDisabled>'
  posFP [m m] : Outport  Port=2  InitialOutput=[0 0]
      settings: AttributesFormatString=initial = '%<InitialOutput>'\nwhen disabled = '%<OutputWhenDisabled>'
  nVec FP [m m] : Outport  Port=3  InitialOutput=0
      settings: AttributesFormatString=initial = '%<InitialOutput>'\nwhen disabled = '%<OutputWhenDisabled>'
  Stiction! : Outport  Port=4  OutputWhenDisabled=reset  InitialOutput=0
      settings: AttributesFormatString=initial = '%<InitialOutput>'\nwhen disabled = '%<OutputWhenDisabled>'
  F_t Slide [N N] : Outport  Port=5  OutputWhenDisabled=reset  InitialOutput=[0 0]
      settings: AttributesFormatString=initial = '%<InitialOutput>'\nwhen disabled = '%<OutputWhenDisabled>'
  F_n Slide [N N] : Outport  Port=6  OutputWhenDisabled=reset  InitialOutput=[0 0]
      settings: AttributesFormatString=initial = '%<InitialOutput>'\nwhen disabled = '%<OutputWhenDisabled>'
  wires:
  RefPt [m m]/1 -> RefPtFP [m m]/1, qnVec/2
  qnVec/1 -> d_n/1
  pos [m m]/1 -> qnVec/1, posFP [m m]/1
  tVec/1 -> reverse direction/1
  Product1/1 -> F_n Slide [N N]/1
  reverse direction/1 -> Scope/1, Product/2
  sliding friction coefficient/1 -> Product/1
  v_nVec/1 -> v_tVec/1
  v_n/1 -> v_nVec/1, Gain4/1
  vel [m/s m/s]/1 -> v_tVec/2, v_n/2
  d_n/1 -> Gain3/1
  nVec [m m]/1 -> nVec FP [m m]/1, Product1/1, d_n/2, v_nVec/2, v_n/1
  Constant/1 -> Sum/2
  Sum/1 -> Negative/1
  Vector Norm/1(norm) -> tVec/2, Sum/1
  Product/1 -> F_t Slide [N N]/1
  Product2/1 -> Product1/2, sliding friction coefficient/1
  Gain3/1 -> Product2/1
  Gain4/1 -> Compare To Constant/1, Add/1
  Constant2/1 -> Add/2
  Compare To Constant/1 -> Product2/3
  Add/1 -> Product2/2
  v_tVec/1 -> Vector Norm/1(vec), tVec/1
  FixPt Relational Operator/1 -> Stiction!/1
  Memory/1 -> FixPt Relational Operator/2
  Negative/1 -> FixPt Relational Operator/1, Memory/1

== system NeuroMuscularLibrary/Ground Contact Model/2D Contact/Static Friction Model ==
  note: Tangential Ground Reaction Force
  note: (distance to
      | surface)
  note: Zero multiplication prevents
      | horizontal friction model from
      | oscillating between static and kinetic
      | friction when the vertical force is zero but
      | the ground level is not yet reached
      | in the upward motion
  note: Static Friction Model
  note: Stiction Limit Detector
  pos [m] : Inport
  vel [m/s m/s] : Inport  Port=2
  RefPtFP [m m] : Inport  Port=3
  posFP [m] : Inport  Port=4
  nVecFP [m m] : Inport  Port=5
  Enable : EnablePort  StatesWhenEnabling=reset  ZeroCross=off
  Abs : Abs
  Add : Sum  Inputs=-+
  Check Vertical Friction : Product  RndMeth=Zero
  Compare To Constant : simulink/Logic and Bit Operations/Compare To Constant  relop=<  const=1  OutDataTypeStr=boolean  ZeroCross=off
  Constant : Constant
  Constant1 : Constant
  D pos_n : DotProduct  InputSameDT=on  OutDataTypeStr=Inherit: Inherit via internal rule
  Dpos_nVec : Product  RndMeth=Zero
  Dpos_tVec : Sum  Inputs=|+-
  FixPt Relational Operator : RelationalOperator  Operator=>  OutDataTypeStr=boolean  ZeroCross=off  RndMeth=Nearest
  Gain : Gain  Gain=-1
  Gain1 : Gain  Gain=k_gn
  Gain2 : Gain  Gain=1/v_gn_max
  Gain3 : Gain  Gain=k_gt
  Gain5 : Gain  Gain=1/v_gt_max
  Memory : Memory
  Positive : simulink/Logic and Bit Operations/Compare To Zero  relop=>  OutDataTypeStr=boolean
  Positive1 : simulink/Logic and Bit Operations/Compare To Zero  relop=>  OutDataTypeStr=boolean
  Product : Product  Inputs=3
  Product1 : Product  RndMeth=Zero
  Sign : Signum  ZeroCross=off
  Sum : Sum  Inputs=-+
  Sum1 : Sum  Inputs=|+-
  Sum2 : Sum  Inputs=|+-
  Vector Norm : Subsystem
  d_n : DotProduct  InputSameDT=on  OutDataTypeStr=Inherit: Inherit via internal rule
  stiction limit force : Gain  Gain=mu_stick
  sum : Sum  Inputs=++|
  tVec1 : Product  Inputs=**  RndMeth=Zero
  tVec2 : Product  Inputs=**  RndMeth=Zero
  v_n : DotProduct  InputSameDT=on  OutDataTypeStr=Inherit: Inherit via internal rule
  v_nVec : Product  RndMeth=Zero
  v_tVec : Sum  Inputs=-+|
  F_n Stick [N N] : Outport  OutputWhenDisabled=reset  InitialOutput=[0 0]
      settings: AttributesFormatString=initial = '%<InitialOutput>'\nwhen disabled = '%<OutputWhenDisabled>'
  F_t Stick [N N] : Outport  Port=2  OutputWhenDisabled=reset  InitialOutput=[0 0]
      settings: AttributesFormatString=when disabled: %<OutputWhenDisabled>\ninitial: %<InitialOutput>
  Sliding! : Outport  Port=3  OutputWhenDisabled=reset  InitialOutput=0
      settings: AttributesFormatString=when disabled: %<OutputWhenDisabled>\ninitial: %<InitialOutput>
  wires:
  Gain5/1 -> tVec1/1
  Sum1/1 -> d_n/2
  RefPtFP [m m]/1 -> Sum1/1
  Vector Norm/1(norm) -> Sum/2
  Gain/1 -> Check Vertical Friction/1
  tVec2/1 -> Gain/1
  sum/1 -> tVec2/1
  Constant/1 -> sum/1
  tVec1/1 -> sum/2
  Sign/1 -> tVec1/2
  Gain3/1 -> tVec2/2, Sign/1
  Dpos_tVec/1 -> Gain3/1
  Dpos_nVec/1 -> Dpos_tVec/2
  D pos_n/1 -> Dpos_nVec/2
  Sum2/1 -> Dpos_tVec/1, D pos_n/2  "Dpos"
  posFP [m]/1 -> Sum2/2
  pos [m]/1 -> Sum1/2, Sum2/1
  Product1/1 -> F_n Stick [N N]/1
  v_tVec/1 -> Gain5/1
  v_nVec/1 -> v_tVec/1
  v_n/1 -> Gain2/1, v_nVec/1
  vel [m/s m/s]/1 -> v_n/1, v_tVec/2
  d_n/1 -> Gain1/1
  nVecFP [m m]/1 -> Product1/1, v_nVec/2, Dpos_nVec/1, D pos_n/1, v_n/2, d_n/1
  Gain1/1 -> Product/1
  Product/1 -> Positive1/1, stiction limit force/1, Product1/2
  Check Vertical Friction/1 -> Vector Norm/1(vec), F_t Stick [N N]/1
  Positive1/1 -> Check Vertical Friction/2
  stiction limit force/1 -> Abs/1
  Abs/1 -> Sum/1
  Sum/1 -> Positive/1
  Gain2/1 -> Compare To Constant/1, Add/1
  Constant1/1 -> Add/2
  Compare To Constant/1 -> Product/3
  Add/1 -> Product/2
  Memory/1 -> FixPt Relational Operator/2
  Positive/1 -> Memory/1, FixPt Relational Operator/1
  FixPt Relational Operator/1 -> Sliding!/1

== system NeuroMuscularLibrary/RMHeel Cnt/3D Contact/Friction Switch ==
  note: Static/Kinetic Friction Switch
  Slide! : Inport
  Stick! : Inport  Port=2
  Memory : Memory
  S-R Flip-Flop : simulink_extras/Flip Flops/S-R Flip-Flop  initial_condition=0
  Terminator : Terminator
  Stiction : Outport
  wires:
  S-R Flip-Flop/1 -> Memory/1
  S-R Flip-Flop/2 -> Terminator/1
  Stick!/1 -> S-R Flip-Flop/1
  Slide!/1 -> S-R Flip-Flop/2
  Memory/1 -> Stiction/1

== system NeuroMuscularLibrary/RMHeel Cnt/3D Contact/Kinetic Friction Model ==
  note: Kinetic Friction Model
  note: Footpoint Determiner
  note: Sliding Limit Detector
  note: Normal Ground Friction
  note: Tangential Ground Friction
  vel [m/s m/s m/s] : Inport
  pos [m m m] : Inport  Port=2
  RefPt [m m m] : Inport  Port=3
  nVec [m m m] : Inport  Port=4
  Enable : EnablePort  StatesWhenEnabling=reset  ZeroCross=off
  Constant : Constant  Value=vLimit
  Constant1 : Constant  Value=[0 0 0 1]'
  Demux : Demux  Outputs=[3 1]
  FixPt Relational Operator : RelationalOperator  Operator=>  OutDataTypeStr=boolean  ZeroCross=off  RndMeth=Nearest
  Gain3 : Gain  Gain=k_gn
  Gain4 : Gain  Gain=1/v_gn_max
  Memory : Memory
  Mux1 : Mux  Inputs=2
  Mux2 : Mux  Inputs=2
  Negative : simulink/Logic and Bit Operations/Compare To Zero  relop=<  OutDataTypeStr=boolean
  Normal Axis Ground Force : Fcn  Expr="u(1)  *  (1-u(2)) * (u(2)<1)"
  Product : Product  RndMeth=Zero
  Product1 : Product  RndMeth=Zero
  Sum : Sum  Inputs=|+-
  Switch : Switch  Criteria=u2 > Threshold  Threshold=0.9*vLimit
      settings: AttributesFormatString=>%<Threshold>?
  Vector Norm : Subsystem
  d_n : DotProduct  InputSameDT=on  OutDataTypeStr=Inherit: Inherit via internal rule
  qnVec : Sum  Inputs=-+
  reverse direction : Gain  Gain=-1
  sliding friction coefficient : Gain  Gain=mu_slide
  tVec : Product  Inputs=*/  RndMeth=Zero
  v_n : DotProduct  InputSameDT=on  OutDataTypeStr=Inherit: Inherit via internal rule
  v_nVec : Product  RndMeth=Zero
  v_tVec : Sum  Inputs=-+|
  RefPtFP [m m m] : Outport  InitialOutput=[0 0 0]
      settings: AttributesFormatString=initial = '%<InitialOutput>'\nwhen disabled = '%<OutputWhenDisabled>'
  posFP [m m m] : Outport  Port=2  InitialOutput=[0 0 0]
      settings: AttributesFormatString=initial = '%<InitialOutput>'\nwhen disabled = '%<OutputWhenDisabled>'
  nVec FP [m m m] : Outport  Port=3  InitialOutput=0
      settings: AttributesFormatString=initial = '%<InitialOutput>'\nwhen disabled = '%<OutputWhenDisabled>'
  Stiction! : Outport  Port=4  OutputWhenDisabled=reset  InitialOutput=0
      settings: AttributesFormatString=initial = '%<InitialOutput>'\nwhen disabled = '%<OutputWhenDisabled>'
  F_t Slide [N N N] : Outport  Port=5  OutputWhenDisabled=reset  InitialOutput=[0 0 0]
      settings: AttributesFormatString=initial = '%<InitialOutput>'\nwhen disabled = '%<OutputWhenDisabled>'
  F_n Slide [N N N] : Outport  Port=6  OutputWhenDisabled=reset  InitialOutput=[0 0 0]
      settings: AttributesFormatString=initial = '%<InitialOutput>'\nwhen disabled = '%<OutputWhenDisabled>'
  wires:
  Normal Axis Ground Force/1 -> sliding friction coefficient/1, Product1/2
  Product/1 -> F_t Slide [N N N]/1
  FixPt Relational Operator/1 -> Stiction!/1
  Memory/1 -> FixPt Relational Operator/2
  Negative/1 -> FixPt Relational Operator/1, Memory/1
  Vector Norm/1(norm) -> Sum/1, Switch/2, Mux2/2
  Sum/1 -> Negative/1
  Constant/1 -> Sum/2
  Mux1/1 -> Normal Axis Ground Force/1
  Gain3/1 -> Mux1/1
  Gain4/1 -> Mux1/2
  nVec [m m m]/1 -> v_n/1, v_nVec/2, d_n/2, Product1/1, nVec FP [m m m]/1
  d_n/1 -> Gain3/1
  vel [m/s m/s m/s]/1 -> v_n/2, v_tVec/2
  v_n/1 -> Gain4/1, v_nVec/1
  v_nVec/1 -> v_tVec/1
  v_tVec/1 -> Vector Norm/1(vec), Mux2/1
  sliding friction coefficient/1 -> Product/1
  reverse direction/1 -> Product/2
  Product1/1 -> F_n Slide [N N N]/1
  tVec/1 -> reverse direction/1
  Constant1/1 -> Switch/3
  Mux2/1 -> Switch/1
  Switch/1 -> Demux/1
  Demux/2 -> tVec/2
  Demux/1 -> tVec/1
  pos [m m m]/1 -> posFP [m m m]/1, qnVec/1
  qnVec/1 -> d_n/1
  RefPt [m m m]/1 -> qnVec/2, RefPtFP [m m m]/1
